simulink model "ControlVehicleVelocity"  (R2020a)
settings: Solver=FixedStepAuto  StartTime=0.0  StopTime=10.0  RelTol=1e-3
PostLoadFcn:
  | config;
undefined symbols (not defined in the file or in its folder): DiscIntNeverNeededParam
libraries: drivingvehiclecontroller x1
settings Model: SimulationMode=software-in-the-loop (sil)  SILPILModeSetting=veronly  Creator=The MathWorks, Inc.  LastModifiedBy=P0158631
settings DataIOCC: ExternalInput=[0, input]  LoadExternalInput=on  ReturnWorkspaceOutputs=off
settings OptimizationCC: DefaultParameterBehavior=Inlined  EnhancedBackFolding=on  PassReuseOutputArgsAs=Individual arguments  ZeroExternalMemoryAtStartup=off  ZeroInternalMemoryAtStartup=off  OptimizeBlockOrder=speed  DifferentSizesBufferReuse=on  OptimizationCustomize=off  EfficientTunableParamExpr=on
settings DebuggingCC: UnderspecifiedInitializationDetection=Classic  MergeDetectMultiDrivingBlocksExec=none  ParameterTunabilityLossMsg=error  ArithmeticOperatorsInVariantConditions=warning
settings HardwareCC: TargetBitPerPointer=64  TargetBitPerSizeT=64  TargetBitPerPtrDiffT=64  TargetLargestAtomicFloat=Float  TargetIntDivRoundTo=Zero  TargetEndianess=LittleEndian  TargetWordSize=64  TargetHWDeviceType=Intel->x86-64 (Windows64)
settings ModelReferenceCC: PropagateSignalLabelsOutOfModel=off
settings SFSimCC: MATLABDynamicMemAlloc=off  CustomCodeUndefinedFunction=UseInterfaceOnly
settings RTWCC: SystemTargetFile=ert.tlc  GenCodeOnly=on  TemplateMakefile=ert_default_tmf  GenerateReport=on
settings CodeAppCC: ForceParamTrailComments=on  IgnoreCustomStorageClasses=off  MaxIdLength=62  OperatorAnnotations=on  SimulinkDataObjDesc=on  SFDataObjDesc=on  InsertBlockDesc=on
settings ERTTargetCC: TargetLangStandard=C99 (ISO)  GenerateSampleERTMain=on  SupportContinuousTime=on  InlinedParameterPlacement=NonHierarchical  ERTCustomFileTemplate=example_file_process.tlc
settings ConfigComp: PSVerificationMode=BugFinder  PSOpenProjectManager=on  PSAddSuffixToResultDir=on  PSAutoStubLUT=on  DVMode=PropertyProving  DVMaxProcessTime=600  DVTestSuiteOptimization=Auto  DVDetectOutOfBounds=on  DVSaveReport=on

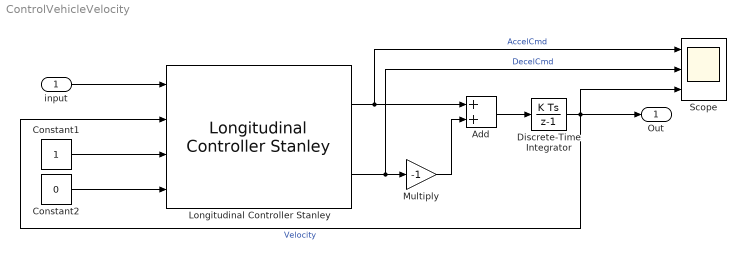
== system ControlVehicleVelocity ==
  input : Inport
  Add : Sum
  Constant1 : Constant
  Constant2 : Constant  Value=0
  Discrete-Time Integrator : DiscreteIntegrator  SampleTime=-1  ICPrevOutput=DiscIntNeverNeededParam  ICPrevScaledInput=DiscIntNeverNeededParam
  Longitudinal Controller Stanley : drivingvehiclecontroller/Longitudinal Controller Stanley  Kp=2.5  Ki=1  SampleTime=0.1  MaxAcceleration=3  MaxDeceleration=6
      link override Verify Direction/Assertion: StopWhenAssertionFail=on
      link override Verify Direction/Assertion1: StopWhenAssertionFail=on
      settings: SourceProductBaseCode=DR
  Multiply : Gain  Gain=-1
  Scope : Scope  NumInputPorts=3
  Out : Outport
  wires:
  Longitudinal Controller Stanley/1 -> Scope/1, Add/1  "AccelCmd"
  Longitudinal Controller Stanley/2 -> Scope/2, Multiply/1  "DecelCmd"
  Multiply/1 -> Add/2
  Add/1 -> Discrete-Time Integrator/1
  Discrete-Time Integrator/1 -> Out/1, Scope/3, Longitudinal Controller Stanley/2  "Velocity"
  input/1 -> Longitudinal Controller Stanley/1
  Constant1/1 -> Longitudinal Controller Stanley/3
  Constant2/1 -> Longitudinal Controller Stanley/4
